simulink model "atrias_system_4khz_with_boom"  (R2016b)
settings: configuration reference "Configuration4khz" (kept outside this file)
undefined symbols (not defined in the file or in its folder): BOOM_MAX_ENCODER_TICKS, elmo_sample_time, gui_disable_cmd, gui_enable_cmd, gui_exit_cmd, gui_reset_cmd, HARD_MOTOR_POSITION_LIMITS_LOWER, HARD_MOTOR_POSITION_LIMITS_UPPER, HIP_ABS_MAX_ENCODER_TICKS, HIP_CURRENT_LIMIT, HIP_INC_MAX_ENCODER_TICKS, HIP_MOTOR_CONSTANT, HIP_MTR_GEAR_RATIO, HIP_MTR_MAX_TORQUE, LEFT_MOTOR_HIP_DIRECTION, LEG1_MOTOR_A_DIRECTION, LEG1_MOTOR_B_DIRECTION, LEG2_MOTOR_A_DIRECTION, LEG2_MOTOR_B_DIRECTION, LEG_CURRENT_LIMIT, LEG_INC_ENCODER_DIRECTION_LEFT_BACK, LEG_INC_ENCODER_DIRECTION_LEFT_FRONT, LEG_INC_ENCODER_DIRECTION_RIGHT_BACK, LEG_INC_ENCODER_DIRECTION_RIGHT_FRONT, LEG_INC_ENCODER_RAD_PER_TICK, LEG_MOTOR_CONSTANT, LEG_MTR_GEAR_RATIO, LEG_MTR_MAX_TORQUE, max_hip_velocity, max_motor_velocity, MEDULLA_ADC_MAX_VOLTS, MEDULLA_ADC_OFFSET_COUNTS, MEDULLA_STATE_ERROR, MEDULLA_STATE_HALT, MEDULLA_STATE_IDLE, MEDULLA_STATE_RESET, MEDULLA_STATE_RUN, MOTOR_POSITION_LIMITS_LOWER, MOTOR_POSITION_LIMITS_UPPER, MTR_HIP_MAX_CURRENT, MTR_MAX_CONT_CURRENT, MTR_MAX_COUNT, MTR_MAX_CURRENT, MTR_MAX_TEMP, RIGHT_MOTOR_HIP_DIRECTION
libraries: xpcethercatlib x203, simulink x38
(part 3 of 4)

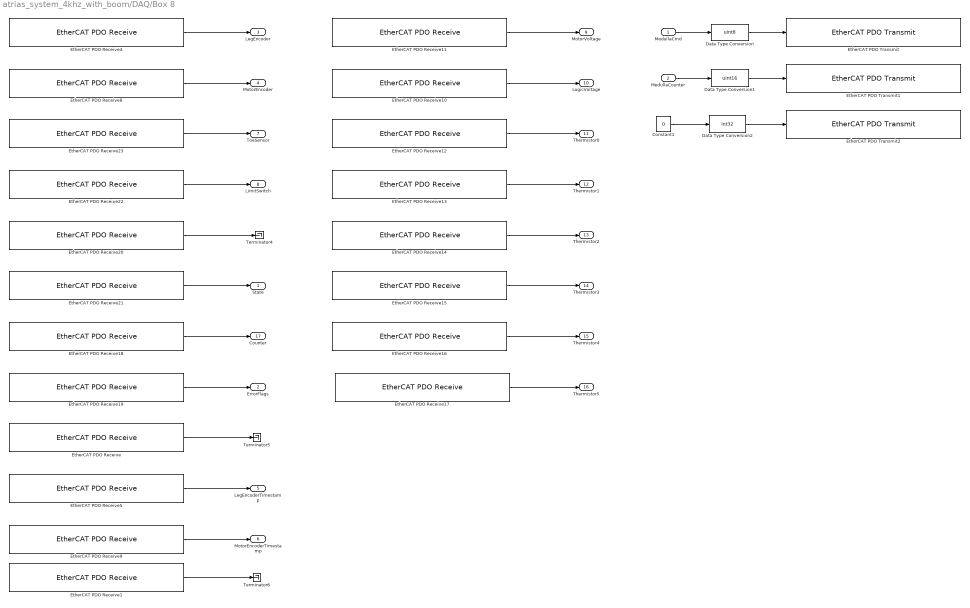
== system atrias_system_4khz_with_boom/DAQ/Box 8 ==
  MedullaCmd : Inport
  MedullaCounter : Inport  Port=2
  Constant1 : Constant  Value=0  OutDataTypeStr=Inherit: Inherit via back propagation
  Data Type Conversion : DataTypeConversion  OutDataTypeStr=uint8
  Data Type Conversion1 : DataTypeConversion  OutDataTypeStr=uint16
  Data Type Conversion2 : DataTypeConversion  OutDataTypeStr=int32
  EtherCAT PDO Receive : xpcethercatlib/EtherCAT PDO Receive  Priority=2  sig_name=Box 8 (ATRIAS 2.1 Leg (Medulla 1.5)).Incremental Encoder.Incremental Encoder  sig_offset=2248  sig_type=uint16  type_size=16  sig_dim=1  device_id=0  sample_time=0.001000
  EtherCAT PDO Receive1 : xpcethercatlib/EtherCAT PDO Receive  Priority=2  sig_name=Box 8 (ATRIAS 2.1 Leg (Medulla 1.5)).Incremental Encoder.Incremental Encoder Timestamp  sig_offset=2264  sig_type=uint16  type_size=16  sig_dim=1  device_id=0  sample_time=0.001000
  EtherCAT PDO Receive10 : xpcethercatlib/EtherCAT PDO Receive  Priority=2  sig_name=Box 8 (ATRIAS 2.1 Leg (Medulla 1.5)).Power.Logic Voltage  sig_offset=2296  sig_type=uint16  type_size=16  sig_dim=1  device_id=0  sample_time=0.001000
  EtherCAT PDO Receive11 : xpcethercatlib/EtherCAT PDO Receive  Priority=2  sig_name=Box 8 (ATRIAS 2.1 Leg (Medulla 1.5)).Power.Motor Voltage  sig_offset=2280  sig_type=uint16  type_size=16  sig_dim=1  device_id=0  sample_time=0.001000
  EtherCAT PDO Receive12 : xpcethercatlib/EtherCAT PDO Receive  Priority=2  sig_name=Box 8 (ATRIAS 2.1 Leg (Medulla 1.5)).Thermistors.Thermistor 0  sig_offset=2312  sig_type=uint16  type_size=16  sig_dim=1  device_id=0  sample_time=0.001000
  EtherCAT PDO Receive13 : xpcethercatlib/EtherCAT PDO Receive  Priority=2  sig_name=Box 8 (ATRIAS 2.1 Leg (Medulla 1.5)).Thermistors.Thermistor 1  sig_offset=2328  sig_type=uint16  type_size=16  sig_dim=1  device_id=0  sample_time=0.001000
  EtherCAT PDO Receive14 : xpcethercatlib/EtherCAT PDO Receive  Priority=2  sig_name=Box 8 (ATRIAS 2.1 Leg (Medulla 1.5)).Thermistors.Thermistor 2  sig_offset=2344  sig_type=uint16  type_size=16  sig_dim=1  device_id=0  sample_time=0.001000
  EtherCAT PDO Receive15 : xpcethercatlib/EtherCAT PDO Receive  Priority=2  sig_name=Box 8 (ATRIAS 2.1 Leg (Medulla 1.5)).Thermistors.Thermistor 3  sig_offset=2360  sig_type=uint16  type_size=16  sig_dim=1  device_id=0  sample_time=0.001000
  EtherCAT PDO Receive16 : xpcethercatlib/EtherCAT PDO Receive  Priority=2  sig_name=Box 8 (ATRIAS 2.1 Leg (Medulla 1.5)).Thermistors.Thermistor 4  sig_offset=2376  sig_type=uint16  type_size=16  sig_dim=1  device_id=0  sample_time=0.001000
  EtherCAT PDO Receive17 : xpcethercatlib/EtherCAT PDO Receive  Priority=2  sig_name=Box 8 (ATRIAS 2.1 Leg (Medulla 1.5)).Thermistors.Thermistor 5  sig_offset=2392  sig_type=uint16  type_size=16  sig_dim=1  device_id=0  sample_time=0.001000
  EtherCAT PDO Receive18 : xpcethercatlib/EtherCAT PDO Receive  Priority=2  sig_name=Box 8 (ATRIAS 2.1 Leg (Medulla 1.5)).uController Status.Counter  sig_offset=2112  sig_type=uint8  type_size=8  sig_dim=1  device_id=0  sample_time=0.001000
  EtherCAT PDO Receive19 : xpcethercatlib/EtherCAT PDO Receive  Priority=2  sig_name=Box 8 (ATRIAS 2.1 Leg (Medulla 1.5)).uController Status.Error Flags  sig_offset=2120  sig_type=uint8  type_size=8  sig_dim=1  device_id=0  sample_time=0.001000
  EtherCAT PDO Receive20 : xpcethercatlib/EtherCAT PDO Receive  Priority=2  sig_name=Box 8 (ATRIAS 2.1 Leg (Medulla 1.5)).uController Status.ID  sig_offset=2096  sig_type=uint8  type_size=8  sig_dim=1  device_id=0  sample_time=0.001000
  EtherCAT PDO Receive21 : xpcethercatlib/EtherCAT PDO Receive  Priority=2  sig_name=Box 8 (ATRIAS 2.1 Leg (Medulla 1.5)).uController Status.State  sig_offset=2104  sig_type=uint8  type_size=8  sig_dim=1  device_id=0  sample_time=0.001000
  EtherCAT PDO Receive22 : xpcethercatlib/EtherCAT PDO Receive  Priority=2  sig_name=Box 8 (ATRIAS 2.1 Leg (Medulla 1.5)).uController Status.Limit Switch  sig_offset=2128  sig_type=uint8  type_size=8  sig_dim=1  device_id=0  sample_time=0.001000
  EtherCAT PDO Receive23 : xpcethercatlib/EtherCAT PDO Receive  Priority=2  sig_name=Box 8 (ATRIAS 2.1 Leg (Medulla 1.5)).uController Status.Toe Sensor  sig_offset=2136  sig_type=uint16  type_size=16  sig_dim=1  device_id=0  sample_time=0.001000
  EtherCAT PDO Receive4 : xpcethercatlib/EtherCAT PDO Receive  Priority=2  sig_name=Box 8 (ATRIAS 2.1 Leg (Medulla 1.5)).Leg Encoder.Leg Encoder  sig_offset=2200  sig_type=uint32  type_size=32  sig_dim=1  device_id=0  sample_time=0.001000
  EtherCAT PDO Receive5 : xpcethercatlib/EtherCAT PDO Receive  Priority=2  sig_name=Box 8 (ATRIAS 2.1 Leg (Medulla 1.5)).Leg Encoder.Leg Encoder Timestamp  sig_offset=2232  sig_type=uint16  type_size=16  sig_dim=1  device_id=0  sample_time=0.001000
  EtherCAT PDO Receive8 : xpcethercatlib/EtherCAT PDO Receive  Priority=2  sig_name=Box 8 (ATRIAS 2.1 Leg (Medulla 1.5)).Motor Encoder.Motor Encoder  sig_offset=2152  sig_type=uint32  type_size=32  sig_dim=1  device_id=0  sample_time=0.001000
  EtherCAT PDO Receive9 : xpcethercatlib/EtherCAT PDO Receive  Priority=2  sig_name=Box 8 (ATRIAS 2.1 Leg (Medulla 1.5)).Motor Encoder.Motor Encoder Timestamp  sig_offset=2184  sig_type=uint16  type_size=16  sig_dim=1  device_id=0  sample_time=0.001000
  EtherCAT PDO Transmit : xpcethercatlib/EtherCAT PDO Transmit   Priority=3  sig_name=Box 8 (ATRIAS 2.1 Leg (Medulla 1.5)).uControllerInput.Command  sig_offset=2096  sig_type=uint8  type_size=8  sig_dim=1  device_id=0  sample_time=0.001000
  EtherCAT PDO Transmit1 : xpcethercatlib/EtherCAT PDO Transmit   Priority=3  sig_name=Box 8 (ATRIAS 2.1 Leg (Medulla 1.5)).uControllerInput.Counter  sig_offset=2104  sig_type=uint16  type_size=16  sig_dim=1  device_id=0  sample_time=0.001000
  EtherCAT PDO Transmit2 : xpcethercatlib/EtherCAT PDO Transmit   Priority=3  sig_name=Box 8 (ATRIAS 2.1 Leg (Medulla 1.5)).uControllerInput.Motor Current  sig_offset=2120  sig_type=int32  type_size=32  sig_dim=1  device_id=0  sample_time=0.001000
  Terminator4 : Terminator
  Terminator5 : Terminator
  Terminator6 : Terminator
  State : Outport
  ErrorFlags : Outport  Port=2
  LegEncoder : Outport  Port=3
  MotorEncoder : Outport  Port=4
  LegEncoderTimestamp : Outport  Port=5
  MotorEncoderTimestamp : Outport  Port=6
  ToeSensor : Outport  Port=7
  LimitSwitch : Outport  Port=8
  MotorVoltage : Outport  Port=9
  LogicVoltage : Outport  Port=10
  Thermistor0 : Outport  Port=11
  Thermistor1 : Outport  Port=12
  Thermistor2 : Outport  Port=13
  Thermistor3 : Outport  Port=14
  Thermistor4 : Outport  Port=15
  Thermistor5 : Outport  Port=16
  Counter : Outport  Port=17
  wires:
  Constant1/1 -> Data Type Conversion2/1
  Data Type Conversion2/1 -> EtherCAT PDO Transmit2/1
  MedullaCounter/1 -> Data Type Conversion1/1
  MedullaCmd/1 -> Data Type Conversion/1
  EtherCAT PDO Receive23/1 -> ToeSensor/1
  EtherCAT PDO Receive21/1 -> State/1
  EtherCAT PDO Receive22/1 -> LimitSwitch/1
  EtherCAT PDO Receive19/1 -> ErrorFlags/1
  EtherCAT PDO Receive18/1 -> Counter/1
  EtherCAT PDO Receive17/1 -> Thermistor5/1
  EtherCAT PDO Receive16/1 -> Thermistor4/1
  EtherCAT PDO Receive15/1 -> Thermistor3/1
  EtherCAT PDO Receive14/1 -> Thermistor2/1
  EtherCAT PDO Receive13/1 -> Thermistor1/1
  EtherCAT PDO Receive12/1 -> Thermistor0/1
  EtherCAT PDO Receive11/1 -> MotorVoltage/1
  EtherCAT PDO Receive10/1 -> LogicVoltage/1
  EtherCAT PDO Receive9/1 -> MotorEncoderTimestamp/1
  EtherCAT PDO Receive8/1 -> MotorEncoder/1
  EtherCAT PDO Receive5/1 -> LegEncoderTimestamp/1
  EtherCAT PDO Receive4/1 -> LegEncoder/1
  EtherCAT PDO Receive1/1 -> Terminator6/1
  EtherCAT PDO Receive/1 -> Terminator5/1
  Data Type Conversion1/1 -> EtherCAT PDO Transmit1/1
  Data Type Conversion/1 -> EtherCAT PDO Transmit/1
  EtherCAT PDO Receive20/1 -> Terminator4/1

== system atrias_system_4khz_with_boom/DAQ/Conversion ==
  note: Convert from Current to Torque
  Elmo Current : Inport
  Constant10 : Constant  Value=LEG_MOTOR_CONSTANT
  Constant11 : Constant  Value=LEG_MTR_GEAR_RATIO
  Convert Elmo PDO to Current : Gain  Gain=MTR_MAX_CONT_CURRENT/1000
  Divide2 : Product  Inputs=****
  LEG1_MOTOR_A_DIRECTION : Constant  Value=LEG1_MOTOR_A_DIRECTION
  LEG1_MOTOR_B_DIRECTION : Constant  Value=LEG1_MOTOR_B_DIRECTION
  LEG2_MOTOR_A_DIRECTION : Constant  Value=LEG2_MOTOR_A_DIRECTION
  LEG2_MOTOR_B_DIRECTION : Constant  Value=LEG2_MOTOR_B_DIRECTION
  Mux2 : Mux
  Torque : Outport
  wires:
  Elmo Current/1 -> Convert Elmo PDO to Current/1
  Constant11/1 -> Divide2/2
  Convert Elmo PDO to Current/1 -> Divide2/3
  Constant10/1 -> Divide2/1
  Divide2/1 -> Torque/1
  LEG1_MOTOR_A_DIRECTION/1 -> Mux2/1
  LEG2_MOTOR_B_DIRECTION/1 -> Mux2/4
  Mux2/1 -> Divide2/4
  LEG2_MOTOR_A_DIRECTION/1 -> Mux2/3
  LEG1_MOTOR_B_DIRECTION/1 -> Mux2/2

== system atrias_system_4khz_with_boom/DAQ/Conversion1 ==
  note: Convert from Current to Torque
  Elmo Current : Inport
  Constant10 : Constant  Value=LEG_MOTOR_CONSTANT
  Constant11 : Constant  Value=LEG_MTR_GEAR_RATIO
  Convert Elmo PDO to Current : Gain  Gain=MTR_MAX_CONT_CURRENT/1000
  Divide2 : Product  Inputs=****
  LEG1_MOTOR_A_DIRECTION : Constant  Value=LEG1_MOTOR_A_DIRECTION
  LEG1_MOTOR_B_DIRECTION : Constant  Value=LEG1_MOTOR_B_DIRECTION
  LEG2_MOTOR_A_DIRECTION : Constant  Value=LEG2_MOTOR_A_DIRECTION
  LEG2_MOTOR_B_DIRECTION : Constant  Value=LEG2_MOTOR_B_DIRECTION
  Mux2 : Mux
  Torque : Outport
  wires:
  LEG1_MOTOR_B_DIRECTION/1 -> Mux2/2
  LEG2_MOTOR_A_DIRECTION/1 -> Mux2/3
  Mux2/1 -> Divide2/4
  LEG2_MOTOR_B_DIRECTION/1 -> Mux2/4
  LEG1_MOTOR_A_DIRECTION/1 -> Mux2/1
  Divide2/1 -> Torque/1
  Constant10/1 -> Divide2/1
  Convert Elmo PDO to Current/1 -> Divide2/3
  Constant11/1 -> Divide2/2
  Elmo Current/1 -> Convert Elmo PDO to Current/1

== system atrias_system_4khz_with_boom/DAQ/Convert geared rad//s to rotor cnts//s ==
  in : Inport
  Gear Ratio : Gain  Gain=LEG_MTR_GEAR_RATIO
  LEG1_MOTOR_A_DIRECTION : Constant  Value=LEG1_MOTOR_A_DIRECTION
  LEG1_MOTOR_B_DIRECTION : Constant  Value=LEG1_MOTOR_B_DIRECTION
  LEG2_MOTOR_A_DIRECTION : Constant  Value=LEG2_MOTOR_A_DIRECTION
  LEG2_MOTOR_B_DIRECTION : Constant  Value=LEG2_MOTOR_B_DIRECTION
  Mux2 : Mux
  Product : Product  RndMeth=Zero
  RadPerSecToCountsPerSec : Gain  Gain=14000/(2*pi)
  out : Outport
  wires:
  RadPerSecToCountsPerSec/1 -> Gear Ratio/1
  in/1 -> RadPerSecToCountsPerSec/1
  LEG1_MOTOR_A_DIRECTION/1 -> Mux2/1
  Product/1 -> out/1
  Gear Ratio/1 -> Product/1
  LEG2_MOTOR_B_DIRECTION/1 -> Mux2/4
  Mux2/1 -> Product/2
  LEG2_MOTOR_A_DIRECTION/1 -> Mux2/3
  LEG1_MOTOR_B_DIRECTION/1 -> Mux2/2

== system atrias_system_4khz_with_boom/DAQ/Convert rotor cnt//s to geared rad//s ==
  in : Inport
  Divide : Product  Inputs=*//
  Gear Ratio : Gain  Gain=LEG_MTR_GEAR_RATIO
  LEG1_MOTOR_A_DIRECTION : Constant  Value=LEG1_MOTOR_A_DIRECTION
  LEG1_MOTOR_B_DIRECTION : Constant  Value=LEG1_MOTOR_B_DIRECTION
  LEG2_MOTOR_A_DIRECTION : Constant  Value=LEG2_MOTOR_A_DIRECTION
  LEG2_MOTOR_B_DIRECTION : Constant  Value=LEG2_MOTOR_B_DIRECTION
  Mux : Mux  Inputs=2
  Mux2 : Mux
  RadPerSecToCountsPerSec : Constant  Value=14000/(2*pi)
  out : Outport
  wires:
  RadPerSecToCountsPerSec/1 -> Gear Ratio/1
  in/1 -> Divide/1
  LEG1_MOTOR_A_DIRECTION/1 -> Mux2/1
  Divide/1 -> out/1
  Gear Ratio/1 -> Divide/2
  LEG2_MOTOR_B_DIRECTION/1 -> Mux2/4
  Mux2/1 -> Mux/1, Mux/2
  LEG2_MOTOR_A_DIRECTION/1 -> Mux2/3
  LEG1_MOTOR_B_DIRECTION/1 -> Mux2/2
  Mux/1 -> Divide/3

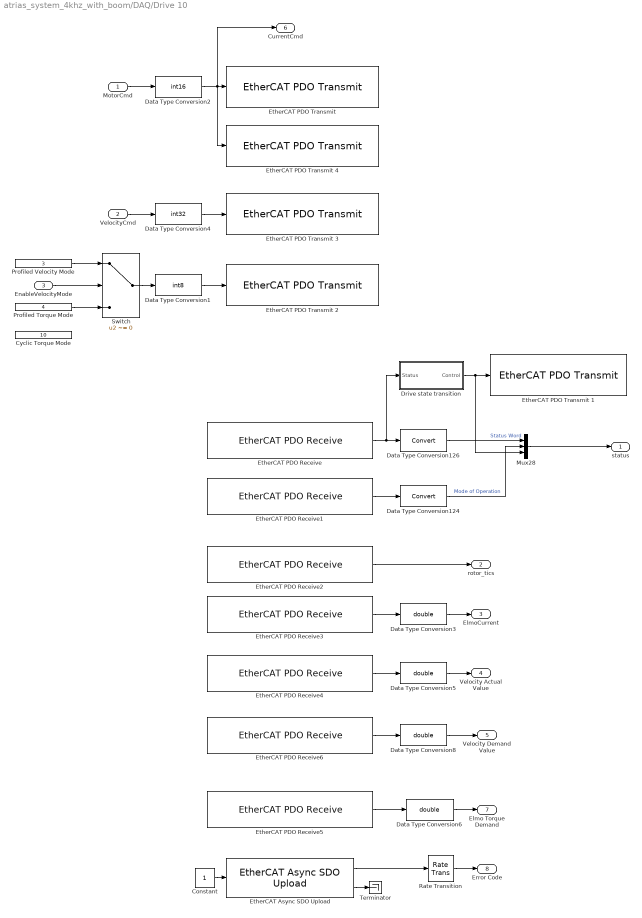
== system atrias_system_4khz_with_boom/DAQ/Drive 10 ==
  MotorCmd : Inport
  VelocityCmd : Inport  Port=2
  EnableVelocityMode : Inport  Port=3
  Constant : Constant  OutDataTypeStr=int32
  Cyclic Torque Mode : Constant  Value=10  OutDataTypeStr=Inherit: Inherit via back propagation
  Data Type Conversion1 : DataTypeConversion  OutDataTypeStr=int8
  Data Type Conversion124 : DataTypeConversion
  Data Type Conversion126 : DataTypeConversion
  Data Type Conversion2 : DataTypeConversion  OutDataTypeStr=int16
  Data Type Conversion{3,5..6,8} (4 alike) : DataTypeConversion  OutDataTypeStr=double
  Data Type Conversion4 : DataTypeConversion  OutDataTypeStr=int32
  Drive state transition : Subsystem
  EtherCAT Async SDO Upload : xpcethercatlib/EtherCAT Async SDO Upload  index=24639  subIndex=0  sig_type=uint16  sig_dim=1  device_id=0  slave_name=Box 10 (Elmo Drive)  sample_time=0.100  slave_addr=1010  selected_slave=Term 1 (EK1100)  timeout=500  slave_found=1
  EtherCAT PDO Receive : xpcethercatlib/EtherCAT PDO Receive  Priority=2  sig_name=Box 10 (Elmo Drive).Inputs.Status word  sig_offset=12976  sig_type=uint16  type_size=16  sig_dim=1  device_id=0  sample_time=0.00025
  EtherCAT PDO Receive1 : xpcethercatlib/EtherCAT PDO Receive  Priority=2  sig_name=Box 10 (Elmo Drive).Inputs.Mode of operation display  sig_offset=12992  sig_type=int8  type_size=8  sig_dim=1  device_id=0  sample_time=0.00025
  EtherCAT PDO Receive2 : xpcethercatlib/EtherCAT PDO Receive  Priority=2  sig_name=Box 10 (Elmo Drive).Inputs.Position actual value  sig_offset=13008  sig_type=int32  type_size=32  sig_dim=1  device_id=0  sample_time=0.00025
  EtherCAT PDO Receive3 : xpcethercatlib/EtherCAT PDO Receive  Priority=2  sig_name=Box 10 (Elmo Drive).Inputs.Current actual value  sig_offset=13120  sig_type=int16  type_size=16  sig_dim=1  device_id=0  sample_time=0.00025
  EtherCAT PDO Receive4 : xpcethercatlib/EtherCAT PDO Receive  Priority=2  sig_name=Box 10 (Elmo Drive).Inputs.Velocity actual value  sig_offset=13072  sig_type=int32  type_size=32  sig_dim=1  device_id=0  sample_time=0.00025
  EtherCAT PDO Receive5 : xpcethercatlib/EtherCAT PDO Receive  Priority=2  sig_name=Box 10 (Elmo Drive).Inputs.Torque demand value  sig_offset=13104  sig_type=int16  type_size=16  sig_dim=1  device_id=0  sample_time=0.00025
  EtherCAT PDO Receive6 : xpcethercatlib/EtherCAT PDO Receive  Priority=2  sig_name=Box 10 (Elmo Drive).Inputs.Velocity demand [cnt/sec]  sig_offset=13040  sig_type=int32  type_size=32  sig_dim=1  device_id=0  sample_time=0.00025
  "EtherCAT PDO Transmit " : xpcethercatlib/EtherCAT PDO Transmit   Priority=3  sig_name=Box 10 (Elmo Drive).Outputs.Target Torque  sig_offset=13008  sig_type=int16  type_size=16  sig_dim=1  device_id=0  sample_time=0.00025
  EtherCAT PDO Transmit 1 : xpcethercatlib/EtherCAT PDO Transmit   Priority=3  sig_name=Box 10 (Elmo Drive).Outputs.Control word  sig_offset=12976  sig_type=uint16  type_size=16  sig_dim=1  device_id=0  sample_time=0.00025
  EtherCAT PDO Transmit 2 : xpcethercatlib/EtherCAT PDO Transmit   Priority=3  sig_name=Box 10 (Elmo Drive).Outputs.Mode of operation  sig_offset=12992  sig_type=int8  type_size=8  sig_dim=1  device_id=0  sample_time=0.00025
  EtherCAT PDO Transmit 3 : xpcethercatlib/EtherCAT PDO Transmit   Priority=3  sig_name=Box 10 (Elmo Drive).Outputs.Target Velocity  sig_offset=13040  sig_type=int32  type_size=32  sig_dim=1  device_id=0  sample_time=0.00025
  EtherCAT PDO Transmit 4 : xpcethercatlib/EtherCAT PDO Transmit   Priority=3  sig_name=Box 10 (Elmo Drive).Outputs.Torque Offset  sig_offset=13024  sig_type=int16  type_size=16  sig_dim=1  device_id=0  sample_time=0.00025
  Mux28 : Mux  Inputs=3
  Profiled Torque Mode : Constant  Value=4  OutDataTypeStr=Inherit: Inherit via back propagation
  Profiled Velocity Mode : Constant  Value=3  OutDataTypeStr=Inherit: Inherit via back propagation
  Rate Transition : RateTransition  Deterministic=off  OutPortSampleTime=sample_time
  Switch : Switch  Criteria=u2 ~= 0
  Terminator : Terminator
  status : Outport
  rotor_tics : Outport  Port=2
  ElmoCurrent : Outport  Port=3
  Velocity Actual Value : Outport  Port=4
  Velocity Demand Value : Outport  Port=5
  CurrentCmd : Outport  Port=6
  Elmo Torque Demand : Outport  Port=7
  Error Code : Outport  Port=8
  wires:
  Data Type Conversion3/1 -> ElmoCurrent/1
  EtherCAT PDO Receive3/1 -> Data Type Conversion3/1
  EtherCAT PDO Receive2/1 -> rotor_tics/1
  Data Type Conversion2/1 -> CurrentCmd/1, EtherCAT PDO Transmit 4/1, "EtherCAT PDO Transmit "/1
  MotorCmd/1 -> Data Type Conversion2/1
  Data Type Conversion1/1 -> EtherCAT PDO Transmit 2/1
  Drive state transition/1(Control) -> EtherCAT PDO Transmit 1/1, Mux28/3
  Switch/1 -> Data Type Conversion1/1
  Data Type Conversion124/1 -> Mux28/2  "Mode of Operation"
  Data Type Conversion126/1 -> Mux28/1  "Status Word"
  Mux28/1 -> status/1
  EtherCAT PDO Receive1/1 -> Data Type Conversion124/1
  EtherCAT PDO Receive/1 -> Drive state transition/1(Status), Data Type Conversion126/1
  Profiled Torque Mode/1 -> Switch/3
  Profiled Velocity Mode/1 -> Switch/1
  EnableVelocityMode/1 -> Switch/2
  Data Type Conversion4/1 -> EtherCAT PDO Transmit 3/1
  VelocityCmd/1 -> Data Type Conversion4/1
  EtherCAT PDO Receive4/1 -> Data Type Conversion5/1
  Data Type Conversion5/1 -> Velocity Actual Value/1
  Data Type Conversion6/1 -> Elmo Torque Demand/1
  EtherCAT PDO Receive5/1 -> Data Type Conversion6/1
  EtherCAT Async SDO Upload/1 -> Rate Transition/1
  Constant/1 -> EtherCAT Async SDO Upload/1
  Rate Transition/1 -> Error Code/1
  EtherCAT Async SDO Upload/2 -> Terminator/1
  EtherCAT PDO Receive6/1 -> Data Type Conversion8/1
  Data Type Conversion8/1 -> Velocity Demand Value/1

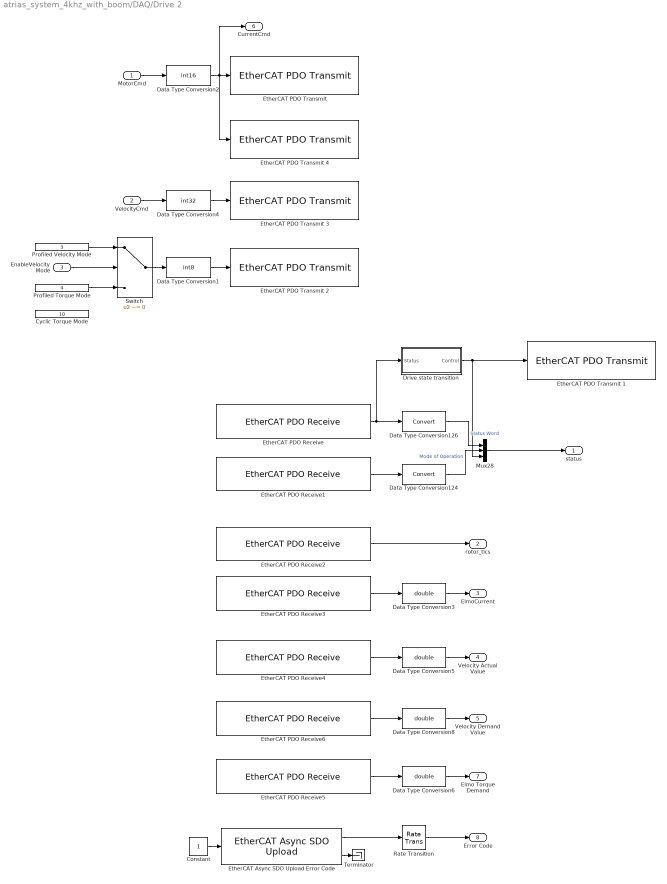
== system atrias_system_4khz_with_boom/DAQ/Drive 2 ==
  MotorCmd : Inport
  VelocityCmd : Inport  Port=2
  EnableVelocity Mode : Inport  Port=3
  Constant : Constant  OutDataTypeStr=int32
  Cyclic Torque Mode : Constant  Value=10  OutDataTypeStr=Inherit: Inherit via back propagation
  Data Type Conversion1 : DataTypeConversion  OutDataTypeStr=int8
  Data Type Conversion124 : DataTypeConversion
  Data Type Conversion126 : DataTypeConversion
  Data Type Conversion2 : DataTypeConversion  OutDataTypeStr=int16
  Data Type Conversion{3,5..6,8} (4 alike) : DataTypeConversion  OutDataTypeStr=double
  Data Type Conversion4 : DataTypeConversion  OutDataTypeStr=int32
  Drive state transition : Subsystem
  EtherCAT Async SDO Upload Error Code : xpcethercatlib/EtherCAT Async SDO Upload  index=24639  subIndex=0  sig_type=uint16  sig_dim=1  device_id=0  slave_name=Box 2 (Elmo Drive)  sample_time=0.100  slave_addr=1002  selected_slave=Term 1 (EK1100)  timeout=500  slave_found=1
  EtherCAT PDO Receive : xpcethercatlib/EtherCAT PDO Receive  Priority=2  sig_name=Box 2 (Elmo Drive).Inputs.Status word  sig_offset=12496  sig_type=uint16  type_size=16  sig_dim=1  device_id=0  sample_time=0.00025
  EtherCAT PDO Receive1 : xpcethercatlib/EtherCAT PDO Receive  Priority=2  sig_name=Box 2 (Elmo Drive).Inputs.Mode of operation display  sig_offset=12512  sig_type=int8  type_size=8  sig_dim=1  device_id=0  sample_time=0.000250
  EtherCAT PDO Receive2 : xpcethercatlib/EtherCAT PDO Receive  Priority=2  sig_name=Box 2 (Elmo Drive).Inputs.Position actual value  sig_offset=12528  sig_type=int32  type_size=32  sig_dim=1  device_id=0  sample_time=0.000250
  EtherCAT PDO Receive3 : xpcethercatlib/EtherCAT PDO Receive  Priority=2  sig_name=Box 2 (Elmo Drive).Inputs.Current actual value  sig_offset=12640  sig_type=int16  type_size=16  sig_dim=1  device_id=0  sample_time=0.000250
  EtherCAT PDO Receive4 : xpcethercatlib/EtherCAT PDO Receive  Priority=2  sig_name=Box 2 (Elmo Drive).Inputs.Velocity actual value  sig_offset=12592  sig_type=int32  type_size=32  sig_dim=1  device_id=0  sample_time=0.000250
  EtherCAT PDO Receive5 : xpcethercatlib/EtherCAT PDO Receive  Priority=2  sig_name=Box 2 (Elmo Drive).Inputs.Torque demand value  sig_offset=12624  sig_type=int16  type_size=16  sig_dim=1  device_id=0  sample_time=0.000250
  EtherCAT PDO Receive6 : xpcethercatlib/EtherCAT PDO Receive  Priority=2  sig_name=Box 2 (Elmo Drive).Inputs.Velocity demand [cnt/sec]  sig_offset=12560  sig_type=int32  type_size=32  sig_dim=1  device_id=0  sample_time=0.000250
  "EtherCAT PDO Transmit " : xpcethercatlib/EtherCAT PDO Transmit   Priority=3  sig_name=Box 2 (Elmo Drive).Outputs.Target Torque  sig_offset=12528  sig_type=int16  type_size=16  sig_dim=1  device_id=0  sample_time=0.000250
  EtherCAT PDO Transmit 1 : xpcethercatlib/EtherCAT PDO Transmit   Priority=3  sig_name=Box 2 (Elmo Drive).Outputs.Control word  sig_offset=12496  sig_type=uint16  type_size=16  sig_dim=1  device_id=0  sample_time=0.000250
  EtherCAT PDO Transmit 2 : xpcethercatlib/EtherCAT PDO Transmit   Priority=3  sig_name=Box 2 (Elmo Drive).Outputs.Mode of operation  sig_offset=12512  sig_type=int8  type_size=8  sig_dim=1  device_id=0  sample_time=0.000250
  EtherCAT PDO Transmit 3 : xpcethercatlib/EtherCAT PDO Transmit   Priority=3  sig_name=Box 2 (Elmo Drive).Outputs.Target Velocity  sig_offset=12560  sig_type=int32  type_size=32  sig_dim=1  device_id=0  sample_time=0.000250
  EtherCAT PDO Transmit 4 : xpcethercatlib/EtherCAT PDO Transmit   Priority=3  sig_name=Box 2 (Elmo Drive).Outputs.Torque Offset  sig_offset=12544  sig_type=int16  type_size=16  sig_dim=1  device_id=0  sample_time=0.000250
  Mux28 : Mux  Inputs=3
  Profiled Torque Mode : Constant  Value=4  OutDataTypeStr=Inherit: Inherit via back propagation
  Profiled Velocity Mode : Constant  Value=3  OutDataTypeStr=Inherit: Inherit via back propagation
  Rate Transition : RateTransition  Deterministic=off  OutPortSampleTime=sample_time
  Switch : Switch  Criteria=u2 ~= 0
  Terminator : Terminator
  status : Outport
  rotor_tics : Outport  Port=2
  ElmoCurrent : Outport  Port=3
  Velocity Actual Value : Outport  Port=4
  Velocity Demand Value : Outport  Port=5
  CurrentCmd : Outport  Port=6
  Elmo Torque Demand : Outport  Port=7
  Error Code : Outport  Port=8
  wires:
  EtherCAT PDO Receive1/1 -> Data Type Conversion124/1
  Mux28/1 -> status/1
  Data Type Conversion126/1 -> Mux28/1  "Status Word"
  Data Type Conversion124/1 -> Mux28/2  "Mode of Operation"
  Drive state transition/1(Control) -> Mux28/3, EtherCAT PDO Transmit 1/1
  EtherCAT PDO Receive2/1 -> rotor_tics/1
  EtherCAT PDO Receive3/1 -> Data Type Conversion3/1
  Data Type Conversion3/1 -> ElmoCurrent/1
  MotorCmd/1 -> Data Type Conversion2/1
  Data Type Conversion1/1 -> EtherCAT PDO Transmit 2/1
  Switch/1 -> Data Type Conversion1/1
  Profiled Torque Mode/1 -> Switch/3
  Profiled Velocity Mode/1 -> Switch/1
  EnableVelocity Mode/1 -> Switch/2
  VelocityCmd/1 -> Data Type Conversion4/1
  Data Type Conversion4/1 -> EtherCAT PDO Transmit 3/1
  EtherCAT PDO Receive4/1 -> Data Type Conversion5/1
  Data Type Conversion5/1 -> Velocity Actual Value/1
  EtherCAT PDO Receive/1 -> Data Type Conversion126/1, Drive state transition/1(Status)
  Data Type Conversion6/1 -> Elmo Torque Demand/1
  EtherCAT PDO Receive5/1 -> Data Type Conversion6/1
  EtherCAT Async SDO Upload Error Code/1 -> Rate Transition/1
  Constant/1 -> EtherCAT Async SDO Upload Error Code/1
  Rate Transition/1 -> Error Code/1
  EtherCAT Async SDO Upload Error Code/2 -> Terminator/1
  EtherCAT PDO Receive6/1 -> Data Type Conversion8/1
  Data Type Conversion8/1 -> Velocity Demand Value/1
  Data Type Conversion2/1 -> EtherCAT PDO Transmit 4/1, CurrentCmd/1, "EtherCAT PDO Transmit "/1

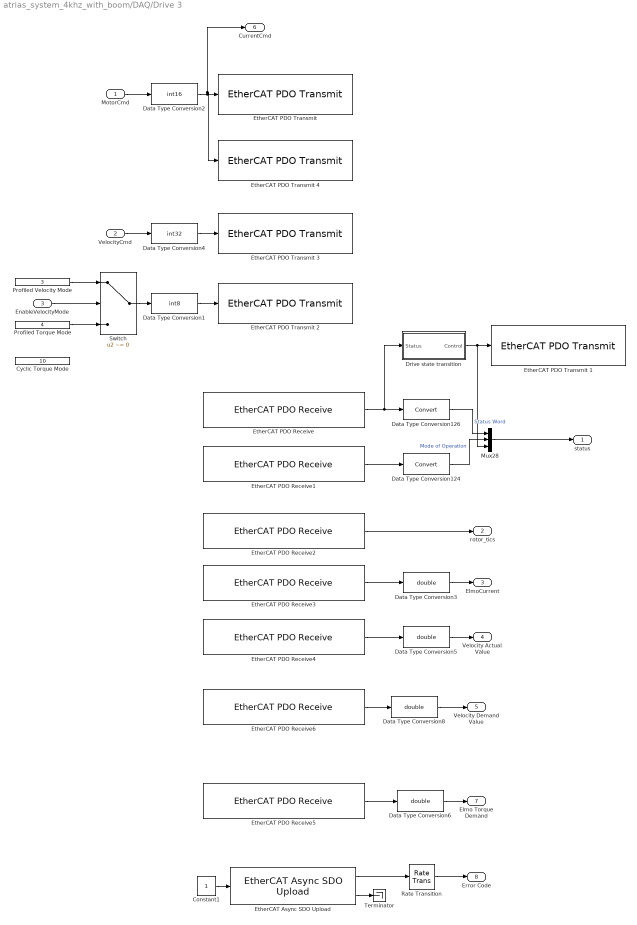
== system atrias_system_4khz_with_boom/DAQ/Drive 3 ==
  MotorCmd : Inport
  VelocityCmd : Inport  Port=2
  EnableVelocityMode : Inport  Port=3
  Constant1 : Constant  OutDataTypeStr=int32
  Cyclic Torque Mode : Constant  Value=10  OutDataTypeStr=Inherit: Inherit via back propagation
  Data Type Conversion1 : DataTypeConversion  OutDataTypeStr=int8
  Data Type Conversion124 : DataTypeConversion
  Data Type Conversion126 : DataTypeConversion
  Data Type Conversion2 : DataTypeConversion  OutDataTypeStr=int16
  Data Type Conversion{3,5..6,8} (4 alike) : DataTypeConversion  OutDataTypeStr=double
  Data Type Conversion4 : DataTypeConversion  OutDataTypeStr=int32
  Drive state transition : Subsystem
  EtherCAT Async SDO Upload : xpcethercatlib/EtherCAT Async SDO Upload  index=24639  subIndex=0  sig_type=uint16  sig_dim=1  device_id=0  slave_name=Box 3 (Elmo Drive)  sample_time=0.100  slave_addr=1003  selected_slave=Term 1 (EK1100)  timeout=500  slave_found=1
  EtherCAT PDO Receive : xpcethercatlib/EtherCAT PDO Receive  Priority=2  sig_name=Box 3 (Elmo Drive).Inputs.Status word  sig_offset=12656  sig_type=uint16  type_size=16  sig_dim=1  device_id=0  sample_time=0.000250
  EtherCAT PDO Receive1 : xpcethercatlib/EtherCAT PDO Receive  Priority=2  sig_name=Box 3 (Elmo Drive).Inputs.Mode of operation display  sig_offset=12672  sig_type=int8  type_size=8  sig_dim=1  device_id=0  sample_time=0.000250
  EtherCAT PDO Receive2 : xpcethercatlib/EtherCAT PDO Receive  Priority=2  sig_name=Box 3 (Elmo Drive).Inputs.Position actual value  sig_offset=12688  sig_type=int32  type_size=32  sig_dim=1  device_id=0  sample_time=0.000250
  EtherCAT PDO Receive3 : xpcethercatlib/EtherCAT PDO Receive  Priority=2  sig_name=Box 3 (Elmo Drive).Inputs.Current actual value  sig_offset=12800  sig_type=int16  type_size=16  sig_dim=1  device_id=0  sample_time=0.000250
  EtherCAT PDO Receive4 : xpcethercatlib/EtherCAT PDO Receive  Priority=2  sig_name=Box 3 (Elmo Drive).Inputs.Velocity actual value  sig_offset=12752  sig_type=int32  type_size=32  sig_dim=1  device_id=0  sample_time=0.000250
  EtherCAT PDO Receive5 : xpcethercatlib/EtherCAT PDO Receive  Priority=2  sig_name=Box 3 (Elmo Drive).Inputs.Torque demand value  sig_offset=12784  sig_type=int16  type_size=16  sig_dim=1  device_id=0  sample_time=0.000250
  EtherCAT PDO Receive6 : xpcethercatlib/EtherCAT PDO Receive  Priority=2  sig_name=Box 3 (Elmo Drive).Inputs.Velocity demand [cnt/sec]  sig_offset=12720  sig_type=int32  type_size=32  sig_dim=1  device_id=0  sample_time=0.000250
  "EtherCAT PDO Transmit " : xpcethercatlib/EtherCAT PDO Transmit   Priority=3  sig_name=Box 3 (Elmo Drive).Outputs.Target Torque  sig_offset=12688  sig_type=int16  type_size=16  sig_dim=1  device_id=0  sample_time=0.000250
  EtherCAT PDO Transmit 1 : xpcethercatlib/EtherCAT PDO Transmit   Priority=3  sig_name=Box 3 (Elmo Drive).Outputs.Control word  sig_offset=12656  sig_type=uint16  type_size=16  sig_dim=1  device_id=0  sample_time=0.000250
  EtherCAT PDO Transmit 2 : xpcethercatlib/EtherCAT PDO Transmit   Priority=3  sig_name=Box 3 (Elmo Drive).Outputs.Mode of operation  sig_offset=12672  sig_type=int8  type_size=8  sig_dim=1  device_id=0  sample_time=0.000250
  EtherCAT PDO Transmit 3 : xpcethercatlib/EtherCAT PDO Transmit   Priority=3  sig_name=Box 3 (Elmo Drive).Outputs.Target Velocity  sig_offset=12720  sig_type=int32  type_size=32  sig_dim=1  device_id=0  sample_time=0.000250
  EtherCAT PDO Transmit 4 : xpcethercatlib/EtherCAT PDO Transmit   Priority=3  sig_name=Box 3 (Elmo Drive).Outputs.Torque Offset  sig_offset=12704  sig_type=int16  type_size=16  sig_dim=1  device_id=0  sample_time=0.000250
  Mux28 : Mux  Inputs=3
  Profiled Torque Mode : Constant  Value=4  OutDataTypeStr=Inherit: Inherit via back propagation
  Profiled Velocity Mode : Constant  Value=3  OutDataTypeStr=Inherit: Inherit via back propagation
  Rate Transition : RateTransition  Deterministic=off  OutPortSampleTime=sample_time
  Switch : Switch  Criteria=u2 ~= 0
  Terminator : Terminator
  status : Outport
  rotor_tics : Outport  Port=2
  ElmoCurrent : Outport  Port=3
  Velocity Actual Value : Outport  Port=4
  Velocity Demand Value : Outport  Port=5
  CurrentCmd : Outport  Port=6
  Elmo Torque Demand : Outport  Port=7
  Error Code : Outport  Port=8
  wires:
  EtherCAT PDO Receive1/1 -> Data Type Conversion124/1
  Mux28/1 -> status/1
  Data Type Conversion126/1 -> Mux28/1  "Status Word"
  Data Type Conversion124/1 -> Mux28/2  "Mode of Operation"
  Drive state transition/1(Control) -> Mux28/3, EtherCAT PDO Transmit 1/1
  EtherCAT PDO Receive2/1 -> rotor_tics/1
  EtherCAT PDO Receive3/1 -> Data Type Conversion3/1
  Data Type Conversion3/1 -> ElmoCurrent/1
  Data Type Conversion2/1 -> EtherCAT PDO Transmit 4/1, CurrentCmd/1, "EtherCAT PDO Transmit "/1
  MotorCmd/1 -> Data Type Conversion2/1
  Data Type Conversion1/1 -> EtherCAT PDO Transmit 2/1
  Switch/1 -> Data Type Conversion1/1
  Profiled Torque Mode/1 -> Switch/3
  Profiled Velocity Mode/1 -> Switch/1
  EnableVelocityMode/1 -> Switch/2
  VelocityCmd/1 -> Data Type Conversion4/1
  Data Type Conversion4/1 -> EtherCAT PDO Transmit 3/1
  EtherCAT PDO Receive4/1 -> Data Type Conversion5/1
  Data Type Conversion5/1 -> Velocity Actual Value/1
  EtherCAT PDO Receive/1 -> Data Type Conversion126/1, Drive state transition/1(Status)
  Data Type Conversion6/1 -> Elmo Torque Demand/1
  EtherCAT PDO Receive5/1 -> Data Type Conversion6/1
  EtherCAT Async SDO Upload/1 -> Rate Transition/1
  Constant1/1 -> EtherCAT Async SDO Upload/1
  Rate Transition/1 -> Error Code/1
  EtherCAT Async SDO Upload/2 -> Terminator/1
  EtherCAT PDO Receive6/1 -> Data Type Conversion8/1
  Data Type Conversion8/1 -> Velocity Demand Value/1

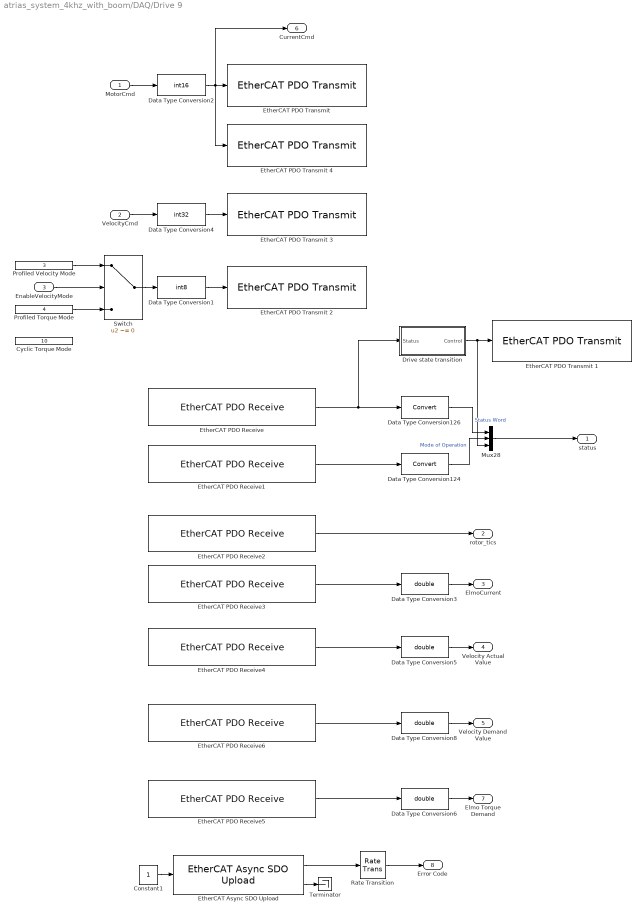
== system atrias_system_4khz_with_boom/DAQ/Drive 9 ==
  MotorCmd : Inport
  VelocityCmd : Inport  Port=2
  EnableVelocityMode : Inport  Port=3
  Constant1 : Constant  OutDataTypeStr=int32
  Cyclic Torque Mode : Constant  Value=10  OutDataTypeStr=Inherit: Inherit via back propagation
  Data Type Conversion1 : DataTypeConversion  OutDataTypeStr=int8
  Data Type Conversion124 : DataTypeConversion
  Data Type Conversion126 : DataTypeConversion
  Data Type Conversion2 : DataTypeConversion  OutDataTypeStr=int16
  Data Type Conversion{3,5..6,8} (4 alike) : DataTypeConversion  OutDataTypeStr=double
  Data Type Conversion4 : DataTypeConversion  OutDataTypeStr=int32
  Drive state transition : Subsystem
  EtherCAT Async SDO Upload : xpcethercatlib/EtherCAT Async SDO Upload  index=24639  subIndex=0  sig_type=uint16  sig_dim=1  device_id=0  slave_name=Box 9 (Elmo Drive)  sample_time=0.100  slave_addr=1009  selected_slave=Term 1 (EK1100)  timeout=500  slave_found=1
  EtherCAT PDO Receive : xpcethercatlib/EtherCAT PDO Receive  Priority=2  sig_name=Box 9 (Elmo Drive).Inputs.Status word  sig_offset=12816  sig_type=uint16  type_size=16  sig_dim=1  device_id=0  sample_time=0.00025
  EtherCAT PDO Receive1 : xpcethercatlib/EtherCAT PDO Receive  Priority=2  sig_name=Box 9 (Elmo Drive).Inputs.Mode of operation display  sig_offset=12832  sig_type=int8  type_size=8  sig_dim=1  device_id=0  sample_time=0.00025
  EtherCAT PDO Receive2 : xpcethercatlib/EtherCAT PDO Receive  Priority=2  sig_name=Box 9 (Elmo Drive).Inputs.Position actual value  sig_offset=12848  sig_type=int32  type_size=32  sig_dim=1  device_id=0  sample_time=0.00025
  EtherCAT PDO Receive3 : xpcethercatlib/EtherCAT PDO Receive  Priority=2  sig_name=Box 9 (Elmo Drive).Inputs.Current actual value  sig_offset=12960  sig_type=int16  type_size=16  sig_dim=1  device_id=0  sample_time=0.00025
  EtherCAT PDO Receive4 : xpcethercatlib/EtherCAT PDO Receive  Priority=2  sig_name=Box 9 (Elmo Drive).Inputs.Velocity actual value  sig_offset=12912  sig_type=int32  type_size=32  sig_dim=1  device_id=0  sample_time=0.00025
  EtherCAT PDO Receive5 : xpcethercatlib/EtherCAT PDO Receive  Priority=2  sig_name=Box 9 (Elmo Drive).Inputs.Torque demand value  sig_offset=12944  sig_type=int16  type_size=16  sig_dim=1  device_id=0  sample_time=0.00025
  EtherCAT PDO Receive6 : xpcethercatlib/EtherCAT PDO Receive  Priority=2  sig_name=Box 9 (Elmo Drive).Inputs.Velocity demand [cnt/sec]  sig_offset=12880  sig_type=int32  type_size=32  sig_dim=1  device_id=0  sample_time=0.00025
  "EtherCAT PDO Transmit " : xpcethercatlib/EtherCAT PDO Transmit   Priority=3  sig_name=Box 9 (Elmo Drive).Outputs.Target Torque  sig_offset=12848  sig_type=int16  type_size=16  sig_dim=1  device_id=0  sample_time=0.00025
  EtherCAT PDO Transmit 1 : xpcethercatlib/EtherCAT PDO Transmit   Priority=3  sig_name=Box 9 (Elmo Drive).Outputs.Control word  sig_offset=12816  sig_type=uint16  type_size=16  sig_dim=1  device_id=0  sample_time=0.00025
  EtherCAT PDO Transmit 2 : xpcethercatlib/EtherCAT PDO Transmit   Priority=3  sig_name=Box 9 (Elmo Drive).Outputs.Mode of operation  sig_offset=12832  sig_type=int8  type_size=8  sig_dim=1  device_id=0  sample_time=0.00025
  EtherCAT PDO Transmit 3 : xpcethercatlib/EtherCAT PDO Transmit   Priority=3  sig_name=Box 9 (Elmo Drive).Outputs.Target Velocity  sig_offset=12880  sig_type=int32  type_size=32  sig_dim=1  device_id=0  sample_time=0.00025
  EtherCAT PDO Transmit 4 : xpcethercatlib/EtherCAT PDO Transmit   Priority=3  sig_name=Box 9 (Elmo Drive).Outputs.Torque Offset  sig_offset=12864  sig_type=int16  type_size=16  sig_dim=1  device_id=0  sample_time=0.00025
  Mux28 : Mux  Inputs=3
  Profiled Torque Mode : Constant  Value=4  OutDataTypeStr=Inherit: Inherit via back propagation
  Profiled Velocity Mode : Constant  Value=3  OutDataTypeStr=Inherit: Inherit via back propagation
  Rate Transition : RateTransition  Deterministic=off  OutPortSampleTime=sample_time
  Switch : Switch  Criteria=u2 ~= 0
  Terminator : Terminator
  status : Outport
  rotor_tics : Outport  Port=2
  ElmoCurrent : Outport  Port=3
  Velocity Actual Value : Outport  Port=4
  Velocity Demand Value : Outport  Port=5
  CurrentCmd : Outport  Port=6
  Elmo Torque Demand : Outport  Port=7
  Error Code : Outport  Port=8
  wires:
  EtherCAT PDO Receive/1 -> Drive state transition/1(Status), Data Type Conversion126/1
  EtherCAT PDO Receive1/1 -> Data Type Conversion124/1
  Mux28/1 -> status/1
  Data Type Conversion126/1 -> Mux28/1  "Status Word"
  Data Type Conversion124/1 -> Mux28/2  "Mode of Operation"
  Drive state transition/1(Control) -> Mux28/3, EtherCAT PDO Transmit 1/1
  EtherCAT PDO Receive2/1 -> rotor_tics/1
  EtherCAT PDO Receive3/1 -> Data Type Conversion3/1
  Data Type Conversion3/1 -> ElmoCurrent/1
  Data Type Conversion2/1 -> CurrentCmd/1, EtherCAT PDO Transmit 4/1, "EtherCAT PDO Transmit "/1
  MotorCmd/1 -> Data Type Conversion2/1
  Data Type Conversion1/1 -> EtherCAT PDO Transmit 2/1
  Switch/1 -> Data Type Conversion1/1
  Profiled Torque Mode/1 -> Switch/3
  Profiled Velocity Mode/1 -> Switch/1
  EnableVelocityMode/1 -> Switch/2
  Data Type Conversion4/1 -> EtherCAT PDO Transmit 3/1
  VelocityCmd/1 -> Data Type Conversion4/1
  EtherCAT PDO Receive4/1 -> Data Type Conversion5/1
  Data Type Conversion5/1 -> Velocity Actual Value/1
  Data Type Conversion6/1 -> Elmo Torque Demand/1
  EtherCAT PDO Receive5/1 -> Data Type Conversion6/1
  EtherCAT Async SDO Upload/1 -> Rate Transition/1
  Constant1/1 -> EtherCAT Async SDO Upload/1
  Rate Transition/1 -> Error Code/1
  EtherCAT Async SDO Upload/2 -> Terminator/1
  EtherCAT PDO Receive6/1 -> Data Type Conversion8/1
  Data Type Conversion8/1 -> Velocity Demand Value/1

== system atrias_system_4khz_with_boom/DAQ/mtr_torque_cmd_to_medulla//elmo_signal ==
  note: Output Order:
      | rB
      | rA
      | lB
      | lA
      | rH
      | lH
  note: Input Order:
      |
      | backR
      | frontR
      | latR
      | backL
      | frontL
      | latL
  tau_cmd [Nm] x6 : Inport
  Constant10 : Constant  Value=LEG_MOTOR_CONSTANT
  Constant11 : Constant  Value=LEG_MTR_GEAR_RATIO
  Constant12 : Constant  Value=HIP_MOTOR_CONSTANT
  Constant13 : Constant  Value=HIP_MTR_GEAR_RATIO
  Constant8 : Constant  Value=MTR_HIP_MAX_CURRENT
  Constant9 : Constant  Value=MTR_MAX_COUNT
  Convert Current to Elmo PDO : Gain  Gain=1000/MTR_MAX_CONT_CURRENT
  Divide1 : Product  Inputs=*/
  Divide2 : Product  Inputs=//*
  Divide3 : Product  Inputs=//*
  Elmo Current Saturation : Saturate  UpperLimit=MTR_MAX_CURRENT  LowerLimit=-MTR_MAX_CURRENT
      settings: AttributesFormatString=Top: %<UpperLimit>\nBottom: %<LowerLimit>
  Hip Motor Current Saturation : Saturate  UpperLimit=MTR_HIP_MAX_CURRENT  LowerLimit=-MTR_HIP_MAX_CURRENT
      settings: AttributesFormatString=Top: %<UpperLimit>\nBottom: %<LowerLimit>
  Hip current limits for testing : Saturate  UpperLimit=HIP_CURRENT_LIMIT  LowerLimit=-HIP_CURRENT_LIMIT
      settings: AttributesFormatString=Top: %<UpperLimit>\nBottom: %<LowerLimit>
  LEFT_MOTOR_HIP_DIRECTION : Constant  Value=LEFT_MOTOR_HIP_DIRECTION
  LEG1_MOTOR_A_DIRECTION : Constant  Value=LEG1_MOTOR_A_DIRECTION
  LEG1_MOTOR_B_DIRECTION : Constant  Value=LEG1_MOTOR_B_DIRECTION
  LEG2_MOTOR_A_DIRECTION : Constant  Value=LEG2_MOTOR_A_DIRECTION
  LEG2_MOTOR_B_DIRECTION : Constant  Value=LEG2_MOTOR_B_DIRECTION
  Lateral Motor Saturation : Saturate  UpperLimit=HIP_MTR_MAX_TORQUE  LowerLimit=-HIP_MTR_MAX_TORQUE
      settings: AttributesFormatString=Top: %<UpperLimit>\nBottom: %<LowerLimit>
  Leg current limits for testing : Saturate  UpperLimit=LEG_CURRENT_LIMIT  LowerLimit=-LEG_CURRENT_LIMIT
      settings: AttributesFormatString=Top: %<UpperLimit>\nBottom: %<LowerLimit>
  Mux : Mux  Inputs=2
  Mux9 : Mux  Inputs=6
  Product : Product  RndMeth=Zero
  Product1 : Product  RndMeth=Zero
  RIGHT_MOTOR_HIP_DIRECTION : Constant  Value=RIGHT_MOTOR_HIP_DIRECTION
  Sagittal Motor Saturation : Saturate  UpperLimit=LEG_MTR_MAX_TORQUE  LowerLimit=-LEG_MTR_MAX_TORQUE
      settings: AttributesFormatString=Top: %<UpperLimit>\nBottom: %<LowerLimit>
  Selector : Selector  InputPortWidth=6  IndexOptions=Index vector (dialog)  Indices=[1 2 4 5 3 6]  OutputSizes=1
  Selector1 : Selector  InputPortWidth=6  IndexOptions=Index vector (dialog)  Indices=[1 2 3 4]  OutputSizes=1
  Selector2 : Selector  InputPortWidth=6  IndexOptions=Index vector (dialog)  Indices=[5 6]  OutputSizes=1
  current_cmd : Outport
  wires:
  Lateral Motor Saturation/1 -> Divide3/3
  Sagittal Motor Saturation/1 -> Divide2/3
  Convert Current to Elmo PDO/1 -> Mux/1
  Mux/1 -> Product/1
  Divide2/1 -> Elmo Current Saturation/1
  Constant12/1 -> Divide3/1
  Constant13/1 -> Divide3/2
  Constant10/1 -> Divide2/1
  Constant11/1 -> Divide2/2
  Selector2/1 -> Lateral Motor Saturation/1  "lateral"
  Selector1/1 -> Sagittal Motor Saturation/1  "sagittal"
  LEG1_MOTOR_A_DIRECTION/1 -> Mux9/1
  LEG1_MOTOR_B_DIRECTION/1 -> Mux9/2
  LEG2_MOTOR_A_DIRECTION/1 -> Mux9/3
  Mux9/1 -> Product/2
  LEG2_MOTOR_B_DIRECTION/1 -> Mux9/4
  RIGHT_MOTOR_HIP_DIRECTION/1 -> Mux9/5
  LEFT_MOTOR_HIP_DIRECTION/1 -> Mux9/6
  Product/1 -> current_cmd/1
  tau_cmd [Nm] x6/1 -> Selector/1
  Selector/1 -> Selector1/1, Selector2/1
  Hip Motor Current Saturation/1 -> Hip current limits for testing/1
  Divide3/1 -> Hip Motor Current Saturation/1
  Constant9/1 -> Divide1/1
  Constant8/1 -> Divide1/2
  Divide1/1 -> Product1/2
  Elmo Current Saturation/1 -> Leg current limits for testing/1
  Product1/1 -> Mux/2
  Hip current limits for testing/1 -> Product1/1
  Leg current limits for testing/1 -> Convert Current to Elmo PDO/1

== system atrias_system_4khz_with_boom/Ramp Velocity Commands/Hold Start Time ==
  Time In : Inport  OutDataTypeStr=double
  Enable : EnablePort
  Time Out : Outport  OutDataTypeStr=double
  wires:
  Time In/1 -> Time Out/1

== system atrias_system_4khz_with_boom/Start Controller/Hold Start Time ==
  Time In : Inport  OutDataTypeStr=double
  Enable : EnablePort
  Time Out : Outport  OutDataTypeStr=double
  wires:
  Time In/1 -> Time Out/1

== system atrias_system_4khz_with_boom/DAQ/Drive 10/Drive state transition ==
  Status : Inport
  Bitwise Operator : simulink/Logic and Bit Operations/Bitwise Operator  logicop=AND  UseBitMask=on  BitMask=hex2dec('ff')  BitMaskRealWorld=Stored Integer
  Bitwise Operator1 : simulink/Logic and Bit Operations/Bitwise Operator  logicop=AND  UseBitMask=on  BitMask=hex2dec('80')  BitMaskRealWorld=Stored Integer
  Compare To Zero : simulink/Logic and Bit Operations/Compare To Zero  relop=~=  OutDataTypeStr=boolean
  Disable Voltage : Constant  Value=0  OutDataTypeStr=uint16
  Fault : simulink/Logic and Bit Operations/Compare To Constant  relop===  const=536  OutDataTypeStr=boolean
  Fault Reset : Constant  Value=128  OutDataTypeStr=uint16
  Fault Reset 2 : Constant  Value=128  OutDataTypeStr=uint16
  Fault reset if warning : Switch  Criteria=u2 > Threshold
  Operation enabled : simulink/Logic and Bit Operations/Compare To Constant  relop===  const=55  OutDataTypeStr=boolean
  Ready to switch ON : simulink/Logic and Bit Operations/Compare To Constant  relop===  const=49  OutDataTypeStr=boolean
  Shutdown : Constant  Value=6  OutDataTypeStr=uint16
  Switch ON : Constant  Value=7  OutDataTypeStr=uint16
  Switch ON Enable Op : Constant  Value=15  OutDataTypeStr=uint16
  Switch ON Enable Op 2 : Constant  Value=15  OutDataTypeStr=uint16
  Switch ON disabled : simulink/Logic and Bit Operations/Compare To Constant  relop===  const=80  OutDataTypeStr=boolean
  Switch{1..5} (5 alike) : Switch  Criteria=u2 > Threshold
  Switched ON : simulink/Logic and Bit Operations/Compare To Constant  relop===  const=51  OutDataTypeStr=boolean
  Control : Outport
  wires:
  Fault Reset 2/1 -> Switch5/1
  Switch5/1 -> Control/1
  Fault/1 -> Switch5/2
  Switch4/1 -> Switch5/3
  Switch ON Enable Op 2/1 -> Switch4/1
  Switch3/1 -> Switch4/3
  Operation enabled/1 -> Switch4/2
  Switch ON Enable Op/1 -> Switch3/1
  Switch2/1 -> Switch3/3
  Switched ON/1 -> Switch3/2
  Switch ON/1 -> Switch2/1
  Switch1/1 -> Switch2/3
  Ready to switch ON/1 -> Switch2/2
  Shutdown/1 -> Switch1/1
  Bitwise Operator/1 -> Switch ON disabled/1, Ready to switch ON/1, Switched ON/1, Operation enabled/1
  Fault reset if warning/1 -> Switch1/3
  Switch ON disabled/1 -> Switch1/2
  Disable Voltage/1 -> Fault reset if warning/3
  Fault Reset/1 -> Fault reset if warning/1
  Compare To Zero/1 -> Fault reset if warning/2
  Bitwise Operator1/1 -> Compare To Zero/1
  Status/1 -> Bitwise Operator/1, Bitwise Operator1/1, Fault/1

== system atrias_system_4khz_with_boom/DAQ/Drive 2/Drive state transition ==
  Status : Inport
  Bitwise Operator : simulink/Logic and Bit Operations/Bitwise Operator  logicop=AND  UseBitMask=on  BitMask=hex2dec('ff')  BitMaskRealWorld=Stored Integer
  Bitwise Operator1 : simulink/Logic and Bit Operations/Bitwise Operator  logicop=AND  UseBitMask=on  BitMask=hex2dec('80')  BitMaskRealWorld=Stored Integer
  Compare To Zero : simulink/Logic and Bit Operations/Compare To Zero  relop=~=  OutDataTypeStr=boolean
  Disable Voltage : Constant  Value=0  OutDataTypeStr=uint16
  Fault : simulink/Logic and Bit Operations/Compare To Constant  relop===  const=536  OutDataTypeStr=boolean
  Fault Reset : Constant  Value=128  OutDataTypeStr=uint16
  Fault Reset 2 : Constant  Value=128  OutDataTypeStr=uint16
  Fault reset if warning : Switch  Criteria=u2 > Threshold
  Operation enabled : simulink/Logic and Bit Operations/Compare To Constant  relop===  const=55  OutDataTypeStr=boolean
  Ready to switch ON : simulink/Logic and Bit Operations/Compare To Constant  relop===  const=49  OutDataTypeStr=boolean
  Shutdown : Constant  Value=6  OutDataTypeStr=uint16
  Switch ON : Constant  Value=7  OutDataTypeStr=uint16
  Switch ON Enable Op : Constant  Value=15  OutDataTypeStr=uint16
  Switch ON Enable Op 2 : Constant  Value=15  OutDataTypeStr=uint16
  Switch ON disabled : simulink/Logic and Bit Operations/Compare To Constant  relop===  const=80  OutDataTypeStr=boolean
  Switch{1..5} (5 alike) : Switch  Criteria=u2 > Threshold
  Switched ON : simulink/Logic and Bit Operations/Compare To Constant  relop===  const=51  OutDataTypeStr=boolean
  Control : Outport
  wires:
  Fault Reset 2/1 -> Switch5/1
  Switch5/1 -> Control/1
  Fault/1 -> Switch5/2
  Switch4/1 -> Switch5/3
  Switch ON Enable Op 2/1 -> Switch4/1
  Switch3/1 -> Switch4/3
  Operation enabled/1 -> Switch4/2
  Switch ON Enable Op/1 -> Switch3/1
  Switch2/1 -> Switch3/3
  Switched ON/1 -> Switch3/2
  Switch ON/1 -> Switch2/1
  Switch1/1 -> Switch2/3
  Ready to switch ON/1 -> Switch2/2
  Shutdown/1 -> Switch1/1
  Bitwise Operator/1 -> Switch ON disabled/1, Ready to switch ON/1, Switched ON/1, Operation enabled/1
  Fault reset if warning/1 -> Switch1/3
  Switch ON disabled/1 -> Switch1/2
  Disable Voltage/1 -> Fault reset if warning/3
  Fault Reset/1 -> Fault reset if warning/1
  Compare To Zero/1 -> Fault reset if warning/2
  Bitwise Operator1/1 -> Compare To Zero/1
  Status/1 -> Bitwise Operator/1, Bitwise Operator1/1, Fault/1

== system atrias_system_4khz_with_boom/DAQ/Drive 3/Drive state transition ==
  Status : Inport
  Bitwise Operator : simulink/Logic and Bit Operations/Bitwise Operator  logicop=AND  UseBitMask=on  BitMask=hex2dec('ff')  BitMaskRealWorld=Stored Integer
  Bitwise Operator1 : simulink/Logic and Bit Operations/Bitwise Operator  logicop=AND  UseBitMask=on  BitMask=hex2dec('80')  BitMaskRealWorld=Stored Integer
  Compare To Zero : simulink/Logic and Bit Operations/Compare To Zero  relop=~=  OutDataTypeStr=boolean
  Disable Voltage : Constant  Value=0  OutDataTypeStr=uint16
  Fault : simulink/Logic and Bit Operations/Compare To Constant  relop===  const=536  OutDataTypeStr=boolean
  Fault Reset : Constant  Value=128  OutDataTypeStr=uint16
  Fault Reset 2 : Constant  Value=128  OutDataTypeStr=uint16
  Fault reset if warning : Switch  Criteria=u2 > Threshold
  Operation enabled : simulink/Logic and Bit Operations/Compare To Constant  relop===  const=55  OutDataTypeStr=boolean
  Ready to switch ON : simulink/Logic and Bit Operations/Compare To Constant  relop===  const=49  OutDataTypeStr=boolean
  Shutdown : Constant  Value=6  OutDataTypeStr=uint16
  Switch ON : Constant  Value=7  OutDataTypeStr=uint16
  Switch ON Enable Op : Constant  Value=15  OutDataTypeStr=uint16
  Switch ON Enable Op 2 : Constant  Value=15  OutDataTypeStr=uint16
  Switch ON disabled : simulink/Logic and Bit Operations/Compare To Constant  relop===  const=80  OutDataTypeStr=boolean
  Switch{1..5} (5 alike) : Switch  Criteria=u2 > Threshold
  Switched ON : simulink/Logic and Bit Operations/Compare To Constant  relop===  const=51  OutDataTypeStr=boolean
  Control : Outport
  wires:
  Fault Reset 2/1 -> Switch5/1
  Switch5/1 -> Control/1
  Fault/1 -> Switch5/2
  Switch4/1 -> Switch5/3
  Switch ON Enable Op 2/1 -> Switch4/1
  Switch3/1 -> Switch4/3
  Operation enabled/1 -> Switch4/2
  Switch ON Enable Op/1 -> Switch3/1
  Switch2/1 -> Switch3/3
  Switched ON/1 -> Switch3/2
  Switch ON/1 -> Switch2/1
  Switch1/1 -> Switch2/3
  Ready to switch ON/1 -> Switch2/2
  Shutdown/1 -> Switch1/1
  Bitwise Operator/1 -> Switch ON disabled/1, Ready to switch ON/1, Switched ON/1, Operation enabled/1
  Fault reset if warning/1 -> Switch1/3
  Switch ON disabled/1 -> Switch1/2
  Disable Voltage/1 -> Fault reset if warning/3
  Fault Reset/1 -> Fault reset if warning/1
  Compare To Zero/1 -> Fault reset if warning/2
  Bitwise Operator1/1 -> Compare To Zero/1
  Status/1 -> Bitwise Operator/1, Bitwise Operator1/1, Fault/1
